simulink model "sample"  (R2020a)
settings: Solver=VariableStepAuto  StartTime=0.0  StopTime=10.0  RelTol=1e-3
settings Model: Creator=Admin  LastModifiedBy=Admin

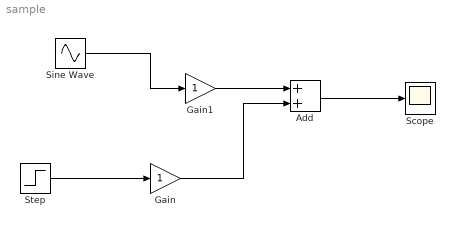
== system sample ==
  Add : Sum
  Gain : Gain
  Gain1 : Gain
  Scope : Scope
  Sine Wave : Sin  SampleTime=0
  Step : Step  SampleTime=0
  wires:
  Step/1 -> Gain/1
  Sine Wave/1 -> Gain1/1
  Add/1 -> Scope/1
  Gain/1 -> Add/2
  Gain1/1 -> Add/1
